simulink model "Y_test"  (R2021a)
settings: Solver=VariableStepAuto  StartTime=0.0  StopTime=10.0  RelTol=1e-3
settings Model: Creator=Zicx  LastModifiedBy=Zicx
settings SolverCC: MaxConsecutiveZCs=1500  ZeroCrossAlgorithm=Adaptive

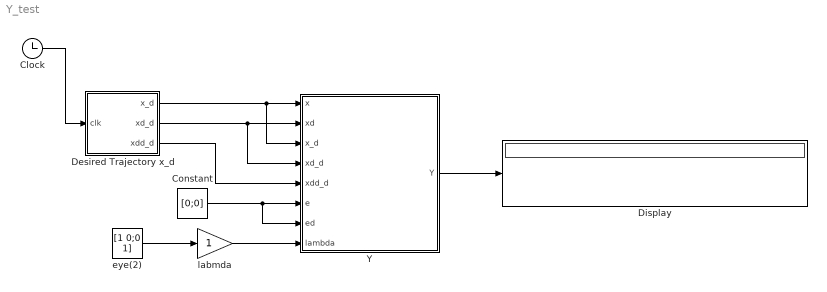
== system Y_test ==
  Clock : Clock
  Constant : Constant  Value=[0;0]  VectorParams1D=off
  Desired Trajectory x_d : Subsystem
  Display : Display
  Y : MATLAB Function  TreatAsAtomicUnit=on
  eye(2) : Constant  Value=[1 0;0 1]  VectorParams1D=off
  labmda : Gain
  wires:
  Clock/1 -> Desired Trajectory x_d/1(clk)
  Desired Trajectory x_d/1(x_d) -> Y/3(x_d), Y/1(x)
  Desired Trajectory x_d/2(xd_d) -> Y/4(xd_d), Y/2(xd)
  Desired Trajectory x_d/3(xdd_d) -> Y/5(xdd_d)
  labmda/1 -> Y/8(lambda)
  eye(2)/1 -> labmda/1
  Y/1(Y) -> Display/1
  Constant/1 -> Y/7(ed), Y/6(e)

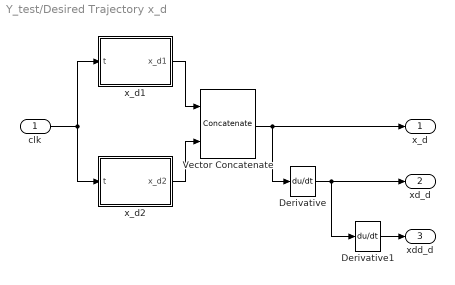
== system Y_test/Desired Trajectory x_d ==
  clk : Inport
  Derivative : Derivative
  Derivative1 : Derivative
  Vector Concatenate : Concatenate
  x_d1 : MATLAB Function  TreatAsAtomicUnit=on
  x_d2 : MATLAB Function  TreatAsAtomicUnit=on
  x_d : Outport
  xd_d : Outport  Port=2
  xdd_d : Outport  Port=3
  wires:
  clk/1 -> x_d2/1(t), x_d1/1(t)
  x_d1/1(x_d1) -> Vector Concatenate/1
  Vector Concatenate/1 -> x_d/1, Derivative/1
  x_d2/1(x_d2) -> Vector Concatenate/2
  Derivative/1 -> Derivative1/1, xd_d/1
  Derivative1/1 -> xdd_d/1

== matlab function Y_test/Desired Trajectory x_d/x_d2 ==
  data: t input; x_d2 output
function x_d2 = fcn(t)

x_d2 = pi/6 * (1 - cos(2 * pi * t) + sin(1.5 * pi * t));

== matlab function Y_test/Desired Trajectory x_d/x_d1 ==
  data: t input; x_d1 output
function x_d1 = fcn(t)

x_d1 = pi/6 * (1 - cos(1.5 * pi * t) + sin(pi * t));

== matlab function Y_test/Y ==
  data: x input; xd input; Y output; x_d input; xd_d input; xdd_d input; e input; ed input; lambda input
function Y = calculateY(x, xd, x_d, xd_d, xdd_d, e, ed, lambda)
Y = system_signals(x, xd, x_d, xd_d, xdd_d, e, ed, lambda);
end
